simulink model "linear_model"  (R2021a)
settings: Solver=VariableStepAuto  StartTime=0.0  StopTime=30  RelTol=1e-3
values from neighbouring files (symbols this model uses):
  A = [-2 0; 1 -3]    [sistemas_lineares.m]
  B = [0.5; 0]    [sistemas_lineares.m]
  C = [0 1]    [sistemas_lineares.m]
  D = 0    [sistemas_lineares.m]
undefined symbols (not defined in the file or in its folder): den, num
settings Model: Creator=Aula  LastModifiedBy=Aula
settings DataIOCC: ReturnWorkspaceOutputs=off

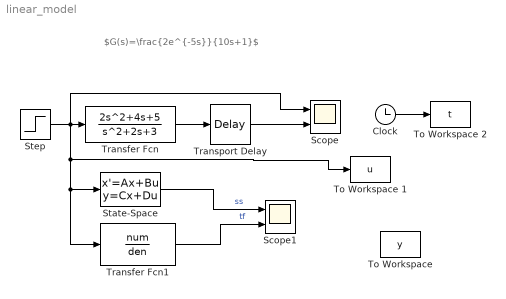
== system linear_model ==
  note: $G(s)=\frac{2e^{-5s}}{10s+1}$
  Clock : Clock
  Scope : Scope  NumInputPorts=2
  Scope1 : Scope  NumInputPorts=2
  State-Space : StateSpace  A=A  B=B  C=C  D=D  InitialCondition=0
  Step : Step  Time=10  SampleTime=0
  "To Workspace " : ToWorkspace  VariableName=y  SampleTime=-1
  To Workspace 1 : ToWorkspace  VariableName=u  SampleTime=-1
  To Workspace 2 : ToWorkspace  VariableName=t  SampleTime=-1
  Transfer Fcn : TransferFcn  Numerator=[2 4 5]  Denominator=[1 2 3]
  Transfer Fcn1 : TransferFcn  Numerator=num  Denominator=den
  Transport Delay : TransportDelay  DelayTime=5
  wires:
  Transfer Fcn/1 -> Transport Delay/1
  Step/1 -> To Workspace 1/1, Transfer Fcn1/1, State-Space/1, Scope/1, Transfer Fcn/1
  Transport Delay/1 -> Scope/2
  Clock/1 -> To Workspace 2/1
  State-Space/1 -> Scope1/1  "ss"
  Transfer Fcn1/1 -> Scope1/2  "tf"
